simulink model "atrias_boom_nmStand_fullCtrl"  (R2015a)
settings: Solver=ode23t  StartTime=0.0  StopTime=t_end  FixedStep=0.001  MaxStep=1e-3  RelTol=1e-3
InitFcn:
  | addpath('../common/')
  | colors
StartFcn:
  | tic
StopFcn:
  | %stopscript
values from neighbouring files (symbols this model uses):
  A1_notch_f1 = -2*cos(fnotch_f1*sample_time)    [set_control_params.m]
  A2_notch_f1 = 1    [set_control_params.m]
  A_lpf_dtau = 1 + B1_lpf_dtau + B2_lpf_dtau    [set_control_params.m]
  ankle_stiffness = 1/2*pi    (= 1.57079632679)    [mechanical_params.m]
  B1_lpf_dtau = -2*exp(-lpf_damping*fcut_dtau*sample_time)*cos(fcut_dtau*sample_time*sqrt(1-lpf_damping^2))    [set_control_params.m]
  B1_notch_f1 = -2*exp(-notch_damping*fnotch_f1*sample_time)*cos(fnotch_f1*sample_time*sqrt(1-notch_damping^2))    [set_control_params.m]
  B2_lpf_dtau = exp(-2*lpf_damping*fcut_dtau*sample_time)    [set_control_params.m]
  B2_notch_f1 = exp(-2*notch_damping*fnotch_f1*sample_time)    [set_control_params.m]
  b_hmotor = 0    [mechanical_params.m]
  b_leg_spring = 0.075*sqrt(k_leg_spring*0.5*.25^2)    [mechanical_params.m]
  b_rotor = 0*60/(2*pi)*9.725e-5    (= 0)    [mechanical_params.m]
  boom_mount_to_center_diagonal = boom_mount_to_center / cos(pitch_mount_angle)    [mechanical_params.m]    (also in set_control_params.m)
  breakaway_friction = [25 25 25 25]    [mechanical_params.m]
  contactThr = 0.35    [set_control_params.m]
  coulomb_friction = [20 20 20 20]    [mechanical_params.m]
  d_com = (d_hip_com_to_torso_com*m_torso)/(m_torso + num_legs*m_hshaft)    [mechanical_params.m]
  delta_phi_max = 160*pi/180    (= 2.79252680319)    [mechanical_params.m]    (also in set_control_params.m)
  delta_phi_max_buffer = 20*pi/180    (= 0.349065850399)    [set_control_params.m]
  delta_phi_max_dropoff = 2*pi/180    (= 0.0349065850399)    [set_control_params.m]
  delta_phi_min = 25.5*pi/180    (= 0.445058959259)    [mechanical_params.m]    (also in set_control_params.m)
  friction_linear_zone = [0.5 0.5 0.5 0.5].*pi/180    [mechanical_params.m]
  g = 9.803    [mechanical_params.m]    (also in set_control_params.m = 9.81)
  gain_nodes_sea_torque = [0,65,350,700]    [set_control_params.m]
  HIP_MTR_MAX_CONT_TORQUE = HIP_MTR_MAX_CONT_CURRENT*HIP_MOTOR_CONSTANT*HIP_MTR_GEAR_RATIO    (= 86.0016)    [set_control_params.m]
  HIP_MTR_MAX_TORQUE = max_current_hip*Kt_hip*N_h    (= 629.28)    [mechanical_params.m]
  initial_boom_pitch = 0    [mechanical_params.m]
  initial_boom_roll = asin((initial_com_height + boom_mount_to_com + boom_mount_to_center*tan(pitch_mount_angle) - (base_12(2) + yshaft_12(2))) / (l_boom + boom_mount_to_center_diagonal))    [mechanical_params.m]
  initial_boom_yaw = 0    [mechanical_params.m]
  initial_hip_roll = 0*pi/180    (= 0)    [mechanical_params.m]
  initial_winch_angle = -12 * pi/180    (= -0.209439510239)    [mechanical_params.m]
  k_gn = m_total*g/0.01    (= 57041.421916)    [mechanical_params.m]
  k_gt = m_total*g/0.1    (= 5704.1421916)    [mechanical_params.m]
  k_leg_spring = 4118.3    [mechanical_params.m]    (also in set_control_params.m)
  K_notch_f1 = (1+B1_notch_f1+B2_notch_f1)/(1+A1_notch_f1+A2_notch_f1)    [set_control_params.m]
  k_phi = 5000    [mechanical_params.m]
  k_sea = [4118.3 4118.3 4118.3 4118.3]    [set_control_params.m]
  Kb_leg = 0.121    [mechanical_params.m]
  kd_boom_roll_Ctrl = 0    [main_1_nmStand.m]    (also in main_2_nmStand_moveBoom.m)
  kd_lateral = 2*sqrt(kp_lateral*0.8)    [set_control_params.m]
  kd_shin_max = kd_pd_avoid_limits    (= 1000)    [set_control_params.m]
  kd_shin_min = kd_pd_avoid_limits    (= 1000)    [set_control_params.m]
  kd_splay_max = kd_pd_avoid_limits    (= 1000)    [set_control_params.m]
  kd_splay_min = kd_pd_avoid_limits    (= 1000)    [set_control_params.m]
  kd_thigh_max = kd_pd_avoid_limits    (= 1000)    [set_control_params.m]
  kd_thigh_min = kd_pd_avoid_limits    (= 1000)    [set_control_params.m]
  kd_winch = td_winch*kp_winch    (= 989.239577798)    [mechanical_params.m]
  kp_boom_roll_Ctrl = 0    [main_1_nmStand.m]    (also in main_2_nmStand_moveBoom.m)
  kp_lateral = 1000    [set_control_params.m]
  kp_sea_torque = [0.3, 0.3, 6.0, 6.0]    [set_control_params.m]
  kp_shin_max = kp_pd_avoid_limits    (= 5000)    [set_control_params.m]
  kp_shin_min = kp_pd_avoid_limits    (= 5000)    [set_control_params.m]
  kp_splay_max = kp_pd_avoid_limits    (= 5000)    [set_control_params.m]
  kp_splay_min = kp_pd_avoid_limits/10    (= 500)    [set_control_params.m]
  kp_thigh_max = kp_pd_avoid_limits    (= 5000)    [set_control_params.m]
  kp_thigh_min = kp_pd_avoid_limits    (= 5000)    [set_control_params.m]
  kp_winch = winch_gravity_comp/(3*pi/180)    (= 19784.791556)    [mechanical_params.m]
  Kt_leg = 0.121    [mechanical_params.m]
  l_boom = 1.8161    [mechanical_params.m]    (also in set_control_params.m)
  L_leg = 0.102e-3    (= 0.000102)    [mechanical_params.m]
  l_seg = 0.5    [mechanical_params.m]    (also in set_control_params.m)
  l_v = l_seg*cos(min_splay_angle/2)    [set_control_params.m]
  lateral_offset = 0.2    [set_control_params.m]
  lateral_target_angle_right = -6*pi/180    (= -0.10471975512)    [set_control_params.m]
  lateral_transition_force = 150    [set_control_params.m]
  LEG_MTR_MAX_TORQUE = max_current_leg * Kt_leg * N    (= 1210)    [mechanical_params.m]
  loaded_unloaded_torque_threshold = 65*ones(1,4)    [set_control_params.m]
  lowerleg_12 = 0.40    (= 0.4)    [mechanical_params.m]
  m_boom = 4.49    [mechanical_params.m]
  m_fblink = 0.46    [mechanical_params.m]    (also in set_control_params.m)
  m_foot = 0.0857    [mechanical_params.m]
  m_hshaft = 18    [mechanical_params.m]    (also in set_control_params.m = 20)
  m_leg = m_thigh + m_lowerleg + m_shin + m_fblink    (= 2.3438)    [mechanical_params.m]
  m_leg_motor = 18    [set_control_params.m]
  m_lowerleg = 0.4438    [mechanical_params.m]    (also in set_control_params.m)
  m_output_gear = 1e-5    (= 1e-05)    [mechanical_params.m]    (also in set_control_params.m)
  m_rotor = 1e-5    (= 1e-05)    [mechanical_params.m]    (also in set_control_params.m)
  m_shin = 0.75    [mechanical_params.m]    (also in set_control_params.m)
  m_thigh = 0.69    [mechanical_params.m]    (also in set_control_params.m)
  m_torso = 17.5    [mechanical_params.m]    (also in set_control_params.m = 17.9)
  m_total = num_legs*(m_hshaft + m_thigh + m_lowerleg + m_shin + m_fblink + 2*m_gearing) + m_torso    (= 58.18772)    [mechanical_params.m]    (also in set_control_params.m = 62.58772)
  m_virtual_gear = 1e-5    (= 1e-05)    [mechanical_params.m]    (also in set_control_params.m)
  m_yshaft = 12.89    [mechanical_params.m]
  max_current_leg = 200    [mechanical_params.m]
  max_sagittal_loaded_torque = 833    [set_control_params.m]
  max_sagittal_unloaded_torque = 267    [set_control_params.m]
  max_torque_lateral = min(MTR_HIP_MAX_CURRENT, HIP_CURRENT_LIMIT)*HIP_MOTOR_CONSTANT*HIP_MTR_GEAR_RATIO    [set_control_params.m]
  max_voltage_leg = 50    [mechanical_params.m]
  maximum_lateral_angle = 18*pi/180    (= 0.314159265359)    [set_control_params.m]
  min_splay_angle = 45*pi/180    (= 0.785398163397)    [set_control_params.m]
  min_splay_buffer = 1*pi/180    (= 0.0174532925199)    [set_control_params.m]
  min_splay_dropoff = 5*pi/180    (= 0.0872664625997)    [set_control_params.m]
  minimum_lateral_angle = -9.5*pi/180    (= -0.165806278939)    [set_control_params.m]
  mu_hmotor = 0.90    (= 0.9)    [mechanical_params.m]
  mu_motor = 0.85    [mechanical_params.m]
  mu_slide = 0.8    [mechanical_params.m]
  mu_stick = 0.9    [mechanical_params.m]
  N = 50    [mechanical_params.m]
  N_h = r_hip_shaft / r_hip_gearhead    (= 57)    [mechanical_params.m]
  phi_max_collision = -5*pi/180    (= -0.0872664625997)    [mechanical_params.m]
  phi_roll_max = pi + 16*pi/180    (= 3.42084533391)    [mechanical_params.m]
  phi_roll_min = pi - 9*pi/180    (= 2.98451302091)    [mechanical_params.m]
  phi_shin_max = 3*pi/2 + 17.5*pi/180    (= 5.01782159948)    [mechanical_params.m]    (also in set_control_params.m)
  phi_shin_max_buffer = 20*pi/180    (= 0.349065850399)    [set_control_params.m]
  phi_shin_max_dropoff = 2*pi/180    (= 0.0349065850399)    [set_control_params.m]
  phi_shin_min = pi - 45*pi/180    (= 2.35619449019)    [mechanical_params.m]    (also in set_control_params.m)
  phi_shin_min_buffer = 20*pi/180    (= 0.349065850399)    [set_control_params.m]
  phi_shin_min_dropoff = 2*pi/180    (= 0.0349065850399)    [set_control_params.m]
  phi_thigh_max = pi + 45*pi/180    (= 3.92699081699)    [mechanical_params.m]    (also in set_control_params.m)
  phi_thigh_max_buffer = 20*pi/180    (= 0.349065850399)    [set_control_params.m]
  phi_thigh_max_dropoff = 2*pi/180    (= 0.0349065850399)    [set_control_params.m]
  phi_thigh_min = pi/2 - 17.5*pi/180    (= 1.2653637077)    [mechanical_params.m]    (also in set_control_params.m)
  phi_thigh_min_buffer = 20*pi/180    (= 0.349065850399)    [set_control_params.m]
  phi_thigh_min_dropoff = 2*pi/180    (= 0.0349065850399)    [set_control_params.m]
  r_hip_gearhead = 0.009525    [mechanical_params.m]
  r_hip_shaft = 0.542925    [mechanical_params.m]
  R_leg = 0.052    [mechanical_params.m]
  r_rotor = 0.001    [mechanical_params.m]
  r_virtual_gear = N*r_rotor    (= 0.05)    [mechanical_params.m]
  releaseThr = 0.2    [set_control_params.m]
  sample_time = 0.001    [set_control_params.m]
  ... (+19 more)
undefined symbols (not defined in the file or in its folder): A_lpf_velocity, B1_lpf_velocity, B2_lpf_velocity, base_color_d, boom_color_d, c, c_jointstop, CtrlPar_theta0, eref, fblink_color_d, floor_color_d, FmaxBFSH, FmaxGLU, FmaxHAM, FmaxHFL, FmaxRF, FmaxVAS, foot_color_d, FPCtrlPar, hshaft_color_d, j_motor, K, lateral_motor_efficiency, LLCtrlPar, loptBFSH, loptGLU, loptHAM, loptHFL, loptRF, loptVAS, lowerleg_color_d, lslackBFSH, lslackGLU, lslackHAM, lslackHFL, lslackRF, lslackVAS, MidDelay_discrete, Newton, output_sample_time, phi12_max, phi12_min, phi23_max, phi23_min, phimaxRFk, phimaxVAS, phirefBFSH, phirefGLU, phirefHAMh, phirefHAMk, phirefHFL, phirefRFh, phirefRFk, phirefVAS, phiScaleRFk, phiScaleVAS, rad ... (+40)
libraries: sm_lib x210, nesl_utility x140, simulink x58, simulink_extras x26, fl_lib x16, mblibv1 x2, commnoisgen2 x1
(part 15 of 19)

== system atrias_boom_nmStand_fullCtrl/Mechanical System Layer/Ground Contact Models/R Back Ground Contact/3D Contact/Static Friction Model ==
  note: Stiction Limit Detector
  note: Static Friction Model
  note: Zero multiplication prevents
      | horizontal friction model from
      | oscillating between static and kinetic
      | friction when the vertical force is zero but
      | the ground level is not yet reached
      | in the upward motion
  note: (distance to
      | surface)
  note: Tangential Ground Reaction Force
  pos [m] : Inport
  vel [m/s m/s m/s] : Inport  Port=2
  RefPtFP [m m m] : Inport  Port=3
  posFP [m] : Inport  Port=4
  nVecFP [m m m] : Inport  Port=5
  Enable : EnablePort  StatesWhenEnabling=reset  ZeroCross=off
  Abs : Abs
  Check Vertical Friction : Product  RndMeth=Zero
  Constant : Constant
  Dpos_n : DotProduct  InputSameDT=on  OutDataTypeStr=Inherit: Inherit via internal rule
  Dpos_nVec : Product  RndMeth=Zero
  Dpos_tVec : Sum  Inputs=|+-
  FixPt Relational Operator : RelationalOperator  Operator=>  OutDataTypeStr=boolean  ZeroCross=off
  Gain : Gain  Gain=-1
  Gain1 : Gain  Gain=k_gn
  Gain2 : Gain  Gain=1/v_gn_max
  Gain3 : Gain  Gain=k_gt
  Gain5 : Gain  Gain=1/v_gt_max
  Memory : Memory
  Mux2 : Mux  Inputs=2
  Normal Ground Reaction Force : Fcn  Expr="u(1)  *  (1-u(2)) * (u(2)<1)"
  Positive : simulink/Logic and Bit Operations/Compare To Zero  relop=>  OutDataTypeStr=boolean
  Positive1 : simulink/Logic and Bit Operations/Compare To Zero  relop=>  OutDataTypeStr=boolean
  Product1 : Product  RndMeth=Zero
  Sign : Signum  ZeroCross=off
  Sum : Sum  Inputs=-+
  Sum1 : Sum  Inputs=|+-
  Sum2 : Sum  Inputs=|+-
  Vector Norm : Subsystem
  d_n : DotProduct  InputSameDT=on  OutDataTypeStr=Inherit: Inherit via internal rule
  stiction limit force : Gain  Gain=mu_stick
  sum : Sum  Inputs=++|
  tVec1 : Product  Inputs=**  RndMeth=Zero
  tVec2 : Product  Inputs=**  RndMeth=Zero
  v_n : DotProduct  InputSameDT=on  OutDataTypeStr=Inherit: Inherit via internal rule
  v_nVec : Product  RndMeth=Zero
  v_tVec : Sum  Inputs=-+|
  F_n Stick [N N N] : Outport  OutputWhenDisabled=reset  InitialOutput=[0 0 0]
      settings: AttributesFormatString=initial = '%<InitialOutput>'\nwhen disabled = '%<OutputWhenDisabled>'
  F_t Stick [N N N] : Outport  Port=2  OutputWhenDisabled=reset  InitialOutput=[0 0 0]
      settings: AttributesFormatString=when disabled: %<OutputWhenDisabled>\ninitial: %<InitialOutput>
  Sliding! : Outport  Port=3  OutputWhenDisabled=reset  InitialOutput=0
      settings: AttributesFormatString=when disabled: %<OutputWhenDisabled>\ninitial: %<InitialOutput>
  wires:
  Sum/1 -> Positive/1
  Memory/1 -> FixPt Relational Operator/2
  Positive/1 -> FixPt Relational Operator/1, Memory/1
  FixPt Relational Operator/1 -> Sliding!/1
  Abs/1 -> Sum/1
  stiction limit force/1 -> Abs/1
  Positive1/1 -> Check Vertical Friction/2
  Check Vertical Friction/1 -> Vector Norm/1(vec), F_t Stick [N N N]/1
  Normal Ground Reaction Force/1 -> Product1/2, stiction limit force/1, Positive1/1
  Mux2/1 -> Normal Ground Reaction Force/1
  Gain1/1 -> Mux2/1
  Gain2/1 -> Mux2/2
  nVecFP [m m m]/1 -> d_n/1, v_n/2, Dpos_n/1, Dpos_nVec/1, v_nVec/2, Product1/1
  d_n/1 -> Gain1/1
  vel [m/s m/s m/s]/1 -> v_tVec/2, v_n/1
  v_n/1 -> v_nVec/1, Gain2/1
  v_nVec/1 -> v_tVec/1
  v_tVec/1 -> Gain5/1
  Product1/1 -> F_n Stick [N N N]/1
  pos [m]/1 -> Sum2/1, Sum1/2
  posFP [m]/1 -> Sum2/2
  Sum2/1 -> Dpos_n/2, Dpos_tVec/1  "Dpos"
  Dpos_n/1 -> Dpos_nVec/2
  Dpos_nVec/1 -> Dpos_tVec/2
  Dpos_tVec/1 -> Gain3/1
  Gain3/1 -> Sign/1, tVec2/2
  Sign/1 -> tVec1/2
  tVec1/1 -> sum/2
  Constant/1 -> sum/1
  sum/1 -> tVec2/1
  tVec2/1 -> Gain/1
  Gain/1 -> Check Vertical Friction/1
  Vector Norm/1(norm) -> Sum/2
  RefPtFP [m m m]/1 -> Sum1/1
  Sum1/1 -> d_n/2
  Gain5/1 -> tVec1/1

== system atrias_boom_nmStand_fullCtrl/Mechanical System Layer/Ground Contact Models/R Front Ground Contact/3D Contact/Friction Switch ==
  note: Static/Kinetic Friction Switch
  Slide! : Inport
  Stick! : Inport  Port=2
  Memory : Memory
  S-R Flip-Flop : simulink_extras/Flip Flops/S-R Flip-Flop  initial_condition=0
  Terminator : Terminator
  Stiction : Outport
  wires:
  S-R Flip-Flop/1 -> Memory/1
  S-R Flip-Flop/2 -> Terminator/1
  Stick!/1 -> S-R Flip-Flop/1
  Slide!/1 -> S-R Flip-Flop/2
  Memory/1 -> Stiction/1

== system atrias_boom_nmStand_fullCtrl/Mechanical System Layer/Ground Contact Models/R Front Ground Contact/3D Contact/Kinetic Friction Model ==
  note: Kinetic Friction Model
  note: Footpoint Determiner
  note: Sliding Limit Detector
  note: Normal Ground Friction
  note: Tangential Ground Friction
  vel [m/s m/s m/s] : Inport
  pos [m m m] : Inport  Port=2
  RefPt [m m m] : Inport  Port=3
  nVec [m m m] : Inport  Port=4
  Enable : EnablePort  StatesWhenEnabling=reset  ZeroCross=off
  Constant : Constant  Value=vLimit
  Constant1 : Constant  Value=[0 0 0 1]'
  Demux : Demux  Outputs=[3 1]
  FixPt Relational Operator : RelationalOperator  Operator=>  OutDataTypeStr=boolean  ZeroCross=off
  Gain3 : Gain  Gain=k_gn
  Gain4 : Gain  Gain=1/v_gn_max
  Memory : Memory
  Mux1 : Mux  Inputs=2
  Mux2 : Mux  Inputs=2
  Negative : simulink/Logic and Bit Operations/Compare To Zero  relop=<  OutDataTypeStr=boolean
  Normal Axis Ground Force : Fcn  Expr="u(1)  *  (1-u(2)) * (u(2)<1)"
  Product : Product  RndMeth=Zero
  Product1 : Product  RndMeth=Zero
  Sum : Sum  Inputs=|+-
  Switch : Switch  Criteria=u2 > Threshold  Threshold=0.9*vLimit
      settings: AttributesFormatString=>%<Threshold>?
  Vector Norm : Subsystem
  d_n : DotProduct  InputSameDT=on  OutDataTypeStr=Inherit: Inherit via internal rule
  qnVec : Sum  Inputs=-+
  reverse direction : Gain  Gain=-1
  sliding friction coefficient : Gain  Gain=mu_slide
  tVec : Product  Inputs=*/  RndMeth=Zero
  v_n : DotProduct  InputSameDT=on  OutDataTypeStr=Inherit: Inherit via internal rule
  v_nVec : Product  RndMeth=Zero
  v_tVec : Sum  Inputs=-+|
  RefPtFP [m m m] : Outport  InitialOutput=[0 0 0]
      settings: AttributesFormatString=initial = '%<InitialOutput>'\nwhen disabled = '%<OutputWhenDisabled>'
  posFP [m m m] : Outport  Port=2  InitialOutput=[0 0 0]
      settings: AttributesFormatString=initial = '%<InitialOutput>'\nwhen disabled = '%<OutputWhenDisabled>'
  nVec FP [m m m] : Outport  Port=3  InitialOutput=0
      settings: AttributesFormatString=initial = '%<InitialOutput>'\nwhen disabled = '%<OutputWhenDisabled>'
  Stiction! : Outport  Port=4  OutputWhenDisabled=reset  InitialOutput=0
      settings: AttributesFormatString=initial = '%<InitialOutput>'\nwhen disabled = '%<OutputWhenDisabled>'
  F_t Slide [N N N] : Outport  Port=5  OutputWhenDisabled=reset  InitialOutput=[0 0 0]
      settings: AttributesFormatString=initial = '%<InitialOutput>'\nwhen disabled = '%<OutputWhenDisabled>'
  F_n Slide [N N N] : Outport  Port=6  OutputWhenDisabled=reset  InitialOutput=[0 0 0]
      settings: AttributesFormatString=initial = '%<InitialOutput>'\nwhen disabled = '%<OutputWhenDisabled>'
  wires:
  Normal Axis Ground Force/1 -> sliding friction coefficient/1, Product1/2
  Product/1 -> F_t Slide [N N N]/1
  FixPt Relational Operator/1 -> Stiction!/1
  Memory/1 -> FixPt Relational Operator/2
  Negative/1 -> FixPt Relational Operator/1, Memory/1
  Vector Norm/1(norm) -> Sum/1, Switch/2, Mux2/2
  Sum/1 -> Negative/1
  Constant/1 -> Sum/2
  Mux1/1 -> Normal Axis Ground Force/1
  Gain3/1 -> Mux1/1
  Gain4/1 -> Mux1/2
  nVec [m m m]/1 -> v_n/1, v_nVec/2, d_n/2, Product1/1, nVec FP [m m m]/1
  d_n/1 -> Gain3/1
  vel [m/s m/s m/s]/1 -> v_n/2, v_tVec/2
  v_n/1 -> Gain4/1, v_nVec/1
  v_nVec/1 -> v_tVec/1
  v_tVec/1 -> Vector Norm/1(vec), Mux2/1
  sliding friction coefficient/1 -> Product/1
  reverse direction/1 -> Product/2
  Product1/1 -> F_n Slide [N N N]/1
  tVec/1 -> reverse direction/1
  Constant1/1 -> Switch/3
  Mux2/1 -> Switch/1
  Switch/1 -> Demux/1
  Demux/2 -> tVec/2
  Demux/1 -> tVec/1
  pos [m m m]/1 -> posFP [m m m]/1, qnVec/1
  qnVec/1 -> d_n/1
  RefPt [m m m]/1 -> qnVec/2, RefPtFP [m m m]/1

== system atrias_boom_nmStand_fullCtrl/Mechanical System Layer/Ground Contact Models/R Front Ground Contact/3D Contact/Static Friction Model ==
  note: Stiction Limit Detector
  note: Static Friction Model
  note: Zero multiplication prevents
      | horizontal friction model from
      | oscillating between static and kinetic
      | friction when the vertical force is zero but
      | the ground level is not yet reached
      | in the upward motion
  note: (distance to
      | surface)
  note: Tangential Ground Reaction Force
  pos [m] : Inport
  vel [m/s m/s m/s] : Inport  Port=2
  RefPtFP [m m m] : Inport  Port=3
  posFP [m] : Inport  Port=4
  nVecFP [m m m] : Inport  Port=5
  Enable : EnablePort  StatesWhenEnabling=reset  ZeroCross=off
  Abs : Abs
  Check Vertical Friction : Product  RndMeth=Zero
  Constant : Constant
  Dpos_n : DotProduct  InputSameDT=on  OutDataTypeStr=Inherit: Inherit via internal rule
  Dpos_nVec : Product  RndMeth=Zero
  Dpos_tVec : Sum  Inputs=|+-
  FixPt Relational Operator : RelationalOperator  Operator=>  OutDataTypeStr=boolean  ZeroCross=off
  Gain : Gain  Gain=-1
  Gain1 : Gain  Gain=k_gn
  Gain2 : Gain  Gain=1/v_gn_max
  Gain3 : Gain  Gain=k_gt
  Gain5 : Gain  Gain=1/v_gt_max
  Memory : Memory
  Mux2 : Mux  Inputs=2
  Normal Ground Reaction Force : Fcn  Expr="u(1)  *  (1-u(2)) * (u(2)<1)"
  Positive : simulink/Logic and Bit Operations/Compare To Zero  relop=>  OutDataTypeStr=boolean
  Positive1 : simulink/Logic and Bit Operations/Compare To Zero  relop=>  OutDataTypeStr=boolean
  Product1 : Product  RndMeth=Zero
  Sign : Signum  ZeroCross=off
  Sum : Sum  Inputs=-+
  Sum1 : Sum  Inputs=|+-
  Sum2 : Sum  Inputs=|+-
  Vector Norm : Subsystem
  d_n : DotProduct  InputSameDT=on  OutDataTypeStr=Inherit: Inherit via internal rule
  stiction limit force : Gain  Gain=mu_stick
  sum : Sum  Inputs=++|
  tVec1 : Product  Inputs=**  RndMeth=Zero
  tVec2 : Product  Inputs=**  RndMeth=Zero
  v_n : DotProduct  InputSameDT=on  OutDataTypeStr=Inherit: Inherit via internal rule
  v_nVec : Product  RndMeth=Zero
  v_tVec : Sum  Inputs=-+|
  F_n Stick [N N N] : Outport  OutputWhenDisabled=reset  InitialOutput=[0 0 0]
      settings: AttributesFormatString=initial = '%<InitialOutput>'\nwhen disabled = '%<OutputWhenDisabled>'
  F_t Stick [N N N] : Outport  Port=2  OutputWhenDisabled=reset  InitialOutput=[0 0 0]
      settings: AttributesFormatString=when disabled: %<OutputWhenDisabled>\ninitial: %<InitialOutput>
  Sliding! : Outport  Port=3  OutputWhenDisabled=reset  InitialOutput=0
      settings: AttributesFormatString=when disabled: %<OutputWhenDisabled>\ninitial: %<InitialOutput>
  wires:
  Sum/1 -> Positive/1
  Memory/1 -> FixPt Relational Operator/2
  Positive/1 -> FixPt Relational Operator/1, Memory/1
  FixPt Relational Operator/1 -> Sliding!/1
  Abs/1 -> Sum/1
  stiction limit force/1 -> Abs/1
  Positive1/1 -> Check Vertical Friction/2
  Check Vertical Friction/1 -> Vector Norm/1(vec), F_t Stick [N N N]/1
  Normal Ground Reaction Force/1 -> Product1/2, stiction limit force/1, Positive1/1
  Mux2/1 -> Normal Ground Reaction Force/1
  Gain1/1 -> Mux2/1
  Gain2/1 -> Mux2/2
  nVecFP [m m m]/1 -> d_n/1, v_n/2, Dpos_n/1, Dpos_nVec/1, v_nVec/2, Product1/1
  d_n/1 -> Gain1/1
  vel [m/s m/s m/s]/1 -> v_tVec/2, v_n/1
  v_n/1 -> v_nVec/1, Gain2/1
  v_nVec/1 -> v_tVec/1
  v_tVec/1 -> Gain5/1
  Product1/1 -> F_n Stick [N N N]/1
  pos [m]/1 -> Sum2/1, Sum1/2
  posFP [m]/1 -> Sum2/2
  Sum2/1 -> Dpos_n/2, Dpos_tVec/1  "Dpos"
  Dpos_n/1 -> Dpos_nVec/2
  Dpos_nVec/1 -> Dpos_tVec/2
  Dpos_tVec/1 -> Gain3/1
  Gain3/1 -> Sign/1, tVec2/2
  Sign/1 -> tVec1/2
  tVec1/1 -> sum/2
  Constant/1 -> sum/1
  sum/1 -> tVec2/1
  tVec2/1 -> Gain/1
  Gain/1 -> Check Vertical Friction/1
  Vector Norm/1(norm) -> Sum/2
  RefPtFP [m m m]/1 -> Sum1/1
  Sum1/1 -> d_n/2
  Gain5/1 -> tVec1/1

== system atrias_boom_nmStand_fullCtrl/Mechanical System Layer/L Leg/Shin SEA/Rotor and Gearing/Rotational Simscape Intf ==
  Ideal Angular Velocity Source : fl_lib/Mechanical/Mechanical Sources/Ideal Angular Velocity Source
  Ideal Torque Sensor : fl_lib/Mechanical/Mechanical Sensors/Ideal Torque Sensor
  w : PMIOPort  Port=1  Side=Left
  T : PMIOPort  Port=2  Side=Right
  R : PMIOPort  Port=3  Side=Left
  C : PMIOPort  Port=4  Side=Right
  connections:
  Ideal Torque Sensor/RConn1 -- C/RConn1
  R/RConn1 -- Ideal Angular Velocity Source/LConn1
  Ideal Torque Sensor/LConn1 -- Ideal Angular Velocity Source/RConn2
  T/RConn1 -- Ideal Torque Sensor/RConn2
  w/RConn1 -- Ideal Angular Velocity Source/RConn1

== system atrias_boom_nmStand_fullCtrl/Mechanical System Layer/L Leg/Thigh SEA/Rotor and Gearing/Rotational Simscape Intf ==
  Ideal Angular Velocity Source : fl_lib/Mechanical/Mechanical Sources/Ideal Angular Velocity Source
  Ideal Torque Sensor : fl_lib/Mechanical/Mechanical Sensors/Ideal Torque Sensor
  w : PMIOPort  Port=1  Side=Left
  T : PMIOPort  Port=2  Side=Right
  R : PMIOPort  Port=3  Side=Left
  C : PMIOPort  Port=4  Side=Right
  connections:
  Ideal Torque Sensor/RConn1 -- C/RConn1
  R/RConn1 -- Ideal Angular Velocity Source/LConn1
  Ideal Torque Sensor/LConn1 -- Ideal Angular Velocity Source/RConn2
  T/RConn1 -- Ideal Torque Sensor/RConn2
  w/RConn1 -- Ideal Angular Velocity Source/RConn1

== system atrias_boom_nmStand_fullCtrl/Mechanical System Layer/R Leg/Shin SEA/Rotor and Gearing/Rotational Simscape Intf ==
  Ideal Angular Velocity Source : fl_lib/Mechanical/Mechanical Sources/Ideal Angular Velocity Source
  Ideal Torque Sensor : fl_lib/Mechanical/Mechanical Sensors/Ideal Torque Sensor
  w : PMIOPort  Port=1  Side=Left
  T : PMIOPort  Port=2  Side=Right
  R : PMIOPort  Port=3  Side=Left
  C : PMIOPort  Port=4  Side=Right
  connections:
  Ideal Torque Sensor/RConn1 -- C/RConn1
  R/RConn1 -- Ideal Angular Velocity Source/LConn1
  Ideal Torque Sensor/LConn1 -- Ideal Angular Velocity Source/RConn2
  T/RConn1 -- Ideal Torque Sensor/RConn2
  w/RConn1 -- Ideal Angular Velocity Source/RConn1

== system atrias_boom_nmStand_fullCtrl/Mechanical System Layer/R Leg/Thigh SEA/Rotor and Gearing/Rotational Simscape Intf ==
  Ideal Angular Velocity Source : fl_lib/Mechanical/Mechanical Sources/Ideal Angular Velocity Source
  Ideal Torque Sensor : fl_lib/Mechanical/Mechanical Sensors/Ideal Torque Sensor
  w : PMIOPort  Port=1  Side=Left
  T : PMIOPort  Port=2  Side=Right
  R : PMIOPort  Port=3  Side=Left
  C : PMIOPort  Port=4  Side=Right
  connections:
  Ideal Torque Sensor/RConn1 -- C/RConn1
  R/RConn1 -- Ideal Angular Velocity Source/LConn1
  Ideal Torque Sensor/LConn1 -- Ideal Angular Velocity Source/RConn2
  T/RConn1 -- Ideal Torque Sensor/RConn2
  w/RConn1 -- Ideal Angular Velocity Source/RConn1

== system atrias_boom_nmStand_fullCtrl/Control/Behavior Control/Add Limit Avoidance PD Torques/mechanical limit avoidance/PD Joint Limit/L Scale desired torque ==
  note: NOTE: min_splay_angle does not equal delta_phi_min
  phi_thigh [rad] : Inport
  phi_shin [rad] : Inport  Port=2
  Constant : Constant
  Constant1 : Constant  Value=delta_phi_max - delta_phi_max_buffer
  Constant10 : Constant  Value=phi_thigh_max_dropoff
  Constant11 : Constant  Value=phi_shin_min_dropoff
  Constant12 : Constant  Value=phi_shin_max_dropoff
  Constant13 : Constant
  Constant2 : Constant  Value=phi_thigh_max - phi_thigh_max_buffer
  Constant3 : Constant  Value=min_splay_angle+min_splay_buffer
  Constant4 : Constant  Value=phi_thigh_min + phi_thigh_min_buffer
  Constant5 : Constant  Value=phi_shin_max - phi_shin_max_buffer
  Constant6 : Constant  Value=phi_shin_min + phi_shin_min_buffer
  Constant7 : Constant  Value=min_splay_dropoff
  Constant8 : Constant  Value=delta_phi_max_dropoff
  Constant9 : Constant  Value=phi_thigh_min_dropoff
  Divide{,1..5} (6 alike) : Product  Inputs=/*
  Gain : Gain  Gain=-1
  Gain1 : Gain  Gain=-1
  Gain2 : Gain  Gain=-1
  L PD scale : Scope  NumInputPorts=4
      settings: ShowLegends=on  TimeRange=2.5  YMin=-100~-5e+07~-1e+07~-5  YMax=100~1e+07~5e+07~5  SaveName=ScopeData5
  Mux{,1,7..8} (4 alike) : Mux  Inputs=2
  Sum : Sum  Inputs=|+-
  Sum1 : Sum  Inputs=-+|
  Sum2 : Sum  Inputs=+-
  Sum{3..8} (6 alike) : Sum  Inputs=+-|
  [0,1]{,1..5} (6 alike) : Saturate  UpperLimit=1  LowerLimit=0
  max : MinMax  Function=max  Inputs=4
  max2 : MinMax  Function=max  Inputs=4
  scale_back : Outport
  scale_front : Outport  Port=2
  wires:
  Mux1/1 -> L PD scale/4
  Sum1/1 -> scale_front/1, Mux1/2
  [min_thigh_scale] -> max2/3
  [max_thigh_scale] -> max2/4
  [max_splay_scale] -> max/4, max2/2
  [min_splay_scale] -> max/3, max2/1
  [max_shin_scale] -> max/2
  [min_shin_scale] -> max/1
  max2/1 -> Sum1/1
  Constant13/1 -> Sum1/2
  Gain2/1 -> Divide5/2
  Constant12/1 -> Divide5/1
  Sum7/1 -> Gain2/1
  "[0,1]5"/1 -> [max_shin_scale]
  Divide5/1 -> "[0,1]5"/1
  Constant11/1 -> Divide4/1
  Sum8/1 -> Divide4/2
  "[0,1]4"/1 -> [min_shin_scale]
  Divide4/1 -> "[0,1]4"/1
  Constant10/1 -> Divide3/1
  Sum5/1 -> Gain1/1
  Gain1/1 -> Divide3/2
  "[0,1]3"/1 -> [max_thigh_scale]
  Divide3/1 -> "[0,1]3"/1
  Constant9/1 -> Divide2/1
  Sum6/1 -> Divide2/2
  "[0,1]2"/1 -> [min_thigh_scale]
  Divide2/1 -> "[0,1]2"/1
  Gain/1 -> Divide1/2
  Constant8/1 -> Divide1/1
  Sum3/1 -> Gain/1
  "[0,1]1"/1 -> [max_splay_scale]
  Divide1/1 -> "[0,1]1"/1
  "[0,1]"/1 -> [min_splay_scale]
  Divide/1 -> "[0,1]"/1
  Sum4/1 -> Divide/2
  Constant7/1 -> Divide/1
  max/1 -> Sum/2
  Constant/1 -> Sum/1
  Sum/1 -> scale_back/1, Mux1/1
  [max_splay_scale] -> Mux7/2  "max_splay_trq"
  [min_splay_scale] -> Mux7/1  "min_splay_trq"
  Mux7/1 -> L PD scale/3
  Mux8/1 -> L PD scale/2
  [max_shin_scale] -> Mux8/2  "max_shin_trq"
  [min_shin_scale] -> Mux8/1  "min_shin_trq"
  Mux/1 -> L PD scale/1
  [max_thigh_scale] -> Mux/2  "max_thigh_trq"
  [min_thigh_scale] -> Mux/1  "min_thigh_trq"
  Constant5/1 -> Sum7/1
  [shin] -> Sum7/2
  Constant6/1 -> Sum8/1
  [shin] -> Sum8/2
  Constant2/1 -> Sum5/1
  [thigh] -> Sum5/2
  Constant4/1 -> Sum6/1
  [thigh] -> Sum6/2
  Constant1/1 -> Sum3/1
  [splay] -> Sum3/2
  Constant3/1 -> Sum4/1
  [splay] -> Sum4/2
  Sum2/1 -> [splay]  "splay angle"
  phi_thigh [rad]/1 -> Sum2/2, [thigh]
  phi_shin [rad]/1 -> Sum2/1, [shin]

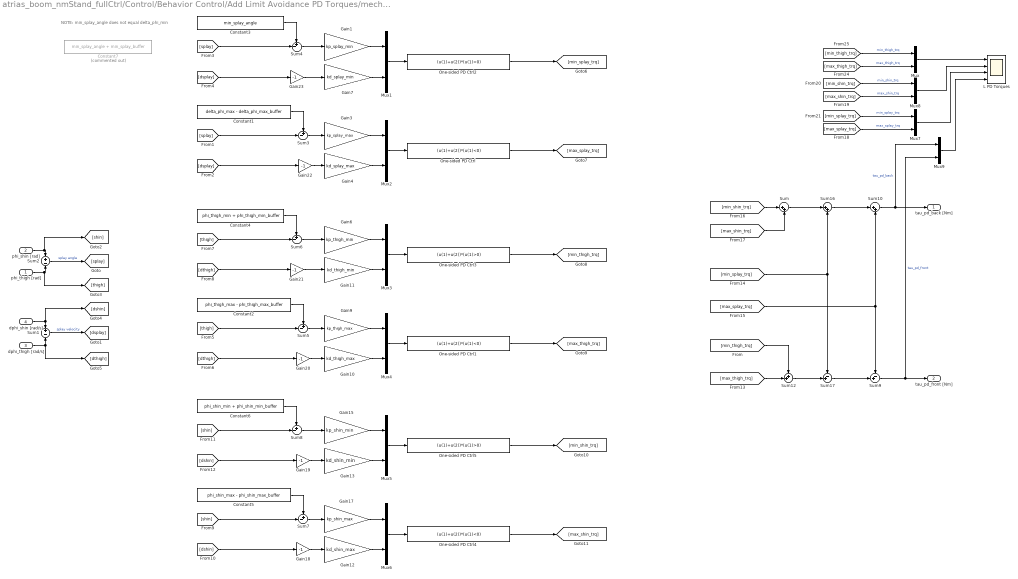
== system atrias_boom_nmStand_fullCtrl/Control/Behavior Control/Add Limit Avoidance PD Torques/mechanical limit avoidance/PD Joint Limit/L mechanical Limit Avoidance Torques (Virtual) ==
  note: NOTE: min_splay_angle does not equal delta_phi_min
  phi_thigh [rad] : Inport
  phi_shin [rad] : Inport  Port=2
  dphi_thigh [rad/s] : Inport  Port=3
  dphi_shin [rad/s] : Inport  Port=4
  Constant1 : Constant  Value=delta_phi_max - delta_phi_max_buffer
  Constant2 : Constant  Value=phi_thigh_max - phi_thigh_max_buffer
  Constant3 : Constant  Value=min_splay_angle
  Constant4 : Constant  Value=phi_thigh_min + phi_thigh_min_buffer
  Constant5 : Constant  Value=phi_shin_max - phi_shin_max_buffer
  Constant6 : Constant  Value=phi_shin_min + phi_shin_min_buffer
  Constant7 : Constant  Commented=on  Value=min_splay_angle + min_splay_buffer
  Gain1 : Gain  Gain=kp_splay_min
  Gain10 : Gain  Gain=kd_thigh_max
  Gain11 : Gain  Gain=kd_thigh_min
  Gain12 : Gain  Gain=kd_shin_max
  Gain13 : Gain  Gain=kd_shin_min
  Gain15 : Gain  Gain=kp_shin_min
  Gain17 : Gain  Gain=kp_shin_max
  Gain{18..23} (6 alike) : Gain  Gain=-1
  Gain3 : Gain  Gain=kp_splay_max
  Gain4 : Gain  Gain=kd_splay_max
  Gain6 : Gain  Gain=kp_thigh_min
  Gain7 : Gain  Gain=kd_splay_min
  Gain9 : Gain  Gain=kp_thigh_max
  L PD Torques : Scope  NumInputPorts=4
      settings: ShowLegends=on  TimeRange=2.5  YMin=-100~-5e+07~-1e+07~-5  YMax=100~1e+07~5e+07~5  SaveName=ScopeData5
  Mux{,1..9} (10 alike) : Mux  Inputs=2
  One-sided PD Ctrl : Fcn  Expr=(u(1)+u(2))*(u(1)<0)
  One-sided PD Ctrl1 : Fcn  Expr=(u(1)+u(2))*(u(1)<0)
  One-sided PD Ctrl2 : Fcn  Expr=(u(1)+u(2))*(u(1)>0)
  One-sided PD Ctrl3 : Fcn  Expr=(u(1)+u(2))*(u(1)>0)
  One-sided PD Ctrl4 : Fcn  Expr=(u(1)+u(2))*(u(1)<0)
  One-sided PD Ctrl5 : Fcn  Expr=(u(1)+u(2))*(u(1)>0)
  Sum : Sum  Inputs=|++
  Sum1 : Sum  Inputs=+-
  Sum10 : Sum  Inputs=|++
  Sum12 : Sum  Inputs=++|
  Sum16 : Sum  Inputs=|++
  Sum17 : Sum  Inputs=-+|
  Sum2 : Sum  Inputs=+-
  Sum{3..8} (6 alike) : Sum  Inputs=+-|
  Sum9 : Sum  Inputs=-+|
  tau_pd_back [Nm] : Outport
  tau_pd_front [Nm] : Outport  Port=2
  wires:
  Mux9/1 -> L PD Torques/4
  dphi_shin [rad/s]/1 -> [dshin], Sum1/1
  dphi_thigh [rad/s]/1 -> [dthigh], Sum1/2
  phi_shin [rad]/1 -> [shin], Sum2/1
  phi_thigh [rad]/1 -> [thigh], Sum2/2
  Sum2/1 -> [splay]  "splay angle"
  Sum1/1 -> [dsplay]  "splay velocity"
  [dsplay] -> Gain23/1
  [splay] -> Sum4/2
  Gain7/1 -> Mux1/2
  Gain1/1 -> Mux1/1
  Sum4/1 -> Gain1/1
  Constant3/1 -> Sum4/1
  Mux1/1 -> One-sided PD Ctrl2/1
  [dsplay] -> Gain22/1
  [splay] -> Sum3/2
  Gain4/1 -> Mux2/2
  Gain3/1 -> Mux2/1
  Sum3/1 -> Gain3/1
  Constant1/1 -> Sum3/1
  Mux2/1 -> One-sided PD Ctrl/1
  [dthigh] -> Gain21/1
  [thigh] -> Sum6/2
  Gain11/1 -> Mux3/2
  Gain6/1 -> Mux3/1
  Sum6/1 -> Gain6/1
  Constant4/1 -> Sum6/1
  Mux3/1 -> One-sided PD Ctrl3/1
  [dthigh] -> Gain20/1
  [thigh] -> Sum5/2
  Gain10/1 -> Mux4/2
  Gain9/1 -> Mux4/1
  Sum5/1 -> Gain9/1
  Constant2/1 -> Sum5/1
  Mux4/1 -> One-sided PD Ctrl1/1
  [dshin] -> Gain19/1
  [shin] -> Sum8/2
  Gain13/1 -> Mux5/2
  Gain15/1 -> Mux5/1
  Sum8/1 -> Gain15/1
  Constant6/1 -> Sum8/1
  Mux5/1 -> One-sided PD Ctrl5/1
  [dshin] -> Gain18/1
  [shin] -> Sum7/2
  Gain12/1 -> Mux6/2
  Gain17/1 -> Mux6/1
  Sum7/1 -> Gain17/1
  Constant5/1 -> Sum7/1
  Mux6/1 -> One-sided PD Ctrl4/1
  One-sided PD Ctrl2/1 -> [min_splay_trq]
  [min_thigh_trq] -> Mux/1  "min_thigh_trq"
  [max_thigh_trq] -> Mux/2  "max_thigh_trq"
  Mux/1 -> L PD Torques/1
  [min_shin_trq] -> Mux8/1  "min_shin_trq"
  [max_shin_trq] -> Mux8/2  "max_shin_trq"
  Mux8/1 -> L PD Torques/2
  Mux7/1 -> L PD Torques/3
  [min_splay_trq] -> Mux7/1  "min_splay_trq"
  [max_splay_trq] -> Mux7/2  "max_splay_trq"
  Sum10/1 -> tau_pd_back [Nm]/1, Mux9/1  "tau_pd_back"
  Sum9/1 -> tau_pd_front [Nm]/1, Mux9/2  "tau_pd_front"
  Sum/1 -> Sum16/1
  [min_shin_trq] -> Sum/1
  [max_shin_trq] -> Sum/2
  Sum16/1 -> Sum10/1
  [min_splay_trq] -> Sum17/1, Sum16/2
  [max_splay_trq] -> Sum9/1, Sum10/2
  [max_thigh_trq] -> Sum12/2
  [min_thigh_trq] -> Sum12/1
  Sum12/1 -> Sum17/2
  Sum17/1 -> Sum9/2
  Gain18/1 -> Gain12/1
  Gain19/1 -> Gain13/1
  Gain20/1 -> Gain10/1
  Gain21/1 -> Gain11/1
  Gain22/1 -> Gain4/1
  Gain23/1 -> Gain7/1
  One-sided PD Ctrl/1 -> [max_splay_trq]
  One-sided PD Ctrl3/1 -> [min_thigh_trq]
  One-sided PD Ctrl1/1 -> [max_thigh_trq]
  One-sided PD Ctrl5/1 -> [min_shin_trq]
  One-sided PD Ctrl4/1 -> [max_shin_trq]

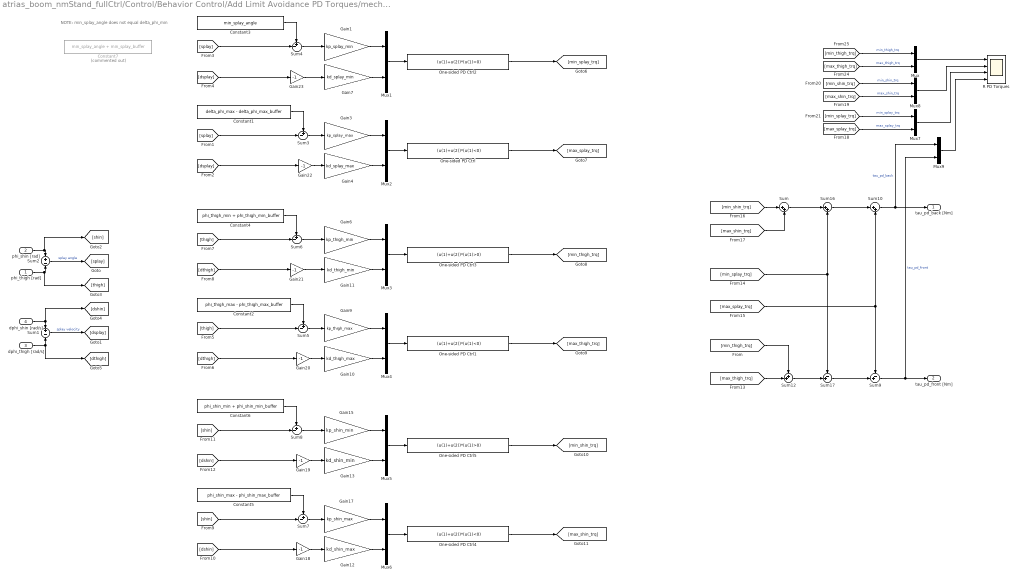
== system atrias_boom_nmStand_fullCtrl/Control/Behavior Control/Add Limit Avoidance PD Torques/mechanical limit avoidance/PD Joint Limit/R Mechanical Limit Avoidance Torques (Virtual)1 ==
  note: NOTE: min_splay_angle does not equal delta_phi_min
  phi_thigh [rad] : Inport
  phi_shin [rad] : Inport  Port=2
  dphi_thigh [rad/s] : Inport  Port=3
  dphi_shin [rad/s] : Inport  Port=4
  Constant1 : Constant  Value=delta_phi_max - delta_phi_max_buffer
  Constant2 : Constant  Value=phi_thigh_max - phi_thigh_max_buffer
  Constant3 : Constant  Value=min_splay_angle
  Constant4 : Constant  Value=phi_thigh_min + phi_thigh_min_buffer
  Constant5 : Constant  Value=phi_shin_max - phi_shin_max_buffer
  Constant6 : Constant  Value=phi_shin_min + phi_shin_min_buffer
  Constant7 : Constant  Commented=on  Value=min_splay_angle + min_splay_buffer
  Gain1 : Gain  Gain=kp_splay_min
  Gain10 : Gain  Gain=kd_thigh_max
  Gain11 : Gain  Gain=kd_thigh_min
  Gain12 : Gain  Gain=kd_shin_max
  Gain13 : Gain  Gain=kd_shin_min
  Gain15 : Gain  Gain=kp_shin_min
  Gain17 : Gain  Gain=kp_shin_max
  Gain{18..23} (6 alike) : Gain  Gain=-1
  Gain3 : Gain  Gain=kp_splay_max
  Gain4 : Gain  Gain=kd_splay_max
  Gain6 : Gain  Gain=kp_thigh_min
  Gain7 : Gain  Gain=kd_splay_min
  Gain9 : Gain  Gain=kp_thigh_max
  Mux{,1..9} (10 alike) : Mux  Inputs=2
  One-sided PD Ctrl : Fcn  Expr=(u(1)+u(2))*(u(1)<0)
  One-sided PD Ctrl1 : Fcn  Expr=(u(1)+u(2))*(u(1)<0)
  One-sided PD Ctrl2 : Fcn  Expr=(u(1)+u(2))*(u(1)>0)
  One-sided PD Ctrl3 : Fcn  Expr=(u(1)+u(2))*(u(1)>0)
  One-sided PD Ctrl4 : Fcn  Expr=(u(1)+u(2))*(u(1)<0)
  One-sided PD Ctrl5 : Fcn  Expr=(u(1)+u(2))*(u(1)>0)
  R PD Torques : Scope  NumInputPorts=4
      settings: ShowLegends=on  TimeRange=2.5  YMin=-100~-5e+07~-1e+07~-5  YMax=100~1e+07~5e+07~5  SaveName=ScopeData5
  Sum : Sum  Inputs=|++
  Sum1 : Sum  Inputs=+-
  Sum10 : Sum  Inputs=|++
  Sum12 : Sum  Inputs=++|
  Sum16 : Sum  Inputs=|++
  Sum17 : Sum  Inputs=-+|
  Sum2 : Sum  Inputs=+-
  Sum{3..8} (6 alike) : Sum  Inputs=+-|
  Sum9 : Sum  Inputs=-+|
  tau_pd_back [Nm] : Outport
  tau_pd_front [Nm] : Outport  Port=2
  wires:
  One-sided PD Ctrl4/1 -> [max_shin_trq]
  One-sided PD Ctrl5/1 -> [min_shin_trq]
  One-sided PD Ctrl1/1 -> [max_thigh_trq]
  One-sided PD Ctrl3/1 -> [min_thigh_trq]
  One-sided PD Ctrl/1 -> [max_splay_trq]
  Gain23/1 -> Gain7/1
  Gain22/1 -> Gain4/1
  Gain21/1 -> Gain11/1
  Gain20/1 -> Gain10/1
  Gain19/1 -> Gain13/1
  Gain18/1 -> Gain12/1
  Sum17/1 -> Sum9/2
  Sum12/1 -> Sum17/2
  [min_thigh_trq] -> Sum12/1
  [max_thigh_trq] -> Sum12/2
  [max_splay_trq] -> Sum10/2, Sum9/1
  [min_splay_trq] -> Sum16/2, Sum17/1
  Sum16/1 -> Sum10/1
  [max_shin_trq] -> Sum/2
  [min_shin_trq] -> Sum/1
  Sum/1 -> Sum16/1
  Sum9/1 -> Mux9/2, tau_pd_front [Nm]/1  "tau_pd_front"
  Sum10/1 -> Mux9/1, tau_pd_back [Nm]/1  "tau_pd_back"
  [max_splay_trq] -> Mux7/2  "max_splay_trq"
  [min_splay_trq] -> Mux7/1  "min_splay_trq"
  Mux7/1 -> R PD Torques/3
  Mux8/1 -> R PD Torques/2
  [max_shin_trq] -> Mux8/2  "max_shin_trq"
  [min_shin_trq] -> Mux8/1  "min_shin_trq"
  Mux/1 -> R PD Torques/1
  [max_thigh_trq] -> Mux/2  "max_thigh_trq"
  [min_thigh_trq] -> Mux/1  "min_thigh_trq"
  One-sided PD Ctrl2/1 -> [min_splay_trq]
  Mux6/1 -> One-sided PD Ctrl4/1
  Constant5/1 -> Sum7/1
  Sum7/1 -> Gain17/1
  Gain17/1 -> Mux6/1
  Gain12/1 -> Mux6/2
  [shin] -> Sum7/2
  [dshin] -> Gain18/1
  Mux5/1 -> One-sided PD Ctrl5/1
  Constant6/1 -> Sum8/1
  Sum8/1 -> Gain15/1
  Gain15/1 -> Mux5/1
  Gain13/1 -> Mux5/2
  [shin] -> Sum8/2
  [dshin] -> Gain19/1
  Mux4/1 -> One-sided PD Ctrl1/1
  Constant2/1 -> Sum5/1
  Sum5/1 -> Gain9/1
  Gain9/1 -> Mux4/1
  Gain10/1 -> Mux4/2
  [thigh] -> Sum5/2
  [dthigh] -> Gain20/1
  Mux3/1 -> One-sided PD Ctrl3/1
  Constant4/1 -> Sum6/1
  Sum6/1 -> Gain6/1
  Gain6/1 -> Mux3/1
  Gain11/1 -> Mux3/2
  [thigh] -> Sum6/2
  [dthigh] -> Gain21/1
  Mux2/1 -> One-sided PD Ctrl/1
  Constant1/1 -> Sum3/1
  Sum3/1 -> Gain3/1
  Gain3/1 -> Mux2/1
  Gain4/1 -> Mux2/2
  [splay] -> Sum3/2
  [dsplay] -> Gain22/1
  Mux1/1 -> One-sided PD Ctrl2/1
  Constant3/1 -> Sum4/1
  Sum4/1 -> Gain1/1
  Gain1/1 -> Mux1/1
  Gain7/1 -> Mux1/2
  [splay] -> Sum4/2
  [dsplay] -> Gain23/1
  Sum1/1 -> [dsplay]  "splay velocity"
  Sum2/1 -> [splay]  "splay angle"
  phi_thigh [rad]/1 -> Sum2/2, [thigh]
  phi_shin [rad]/1 -> Sum2/1, [shin]
  dphi_thigh [rad/s]/1 -> Sum1/2, [dthigh]
  dphi_shin [rad/s]/1 -> Sum1/1, [dshin]
  Mux9/1 -> R PD Torques/4

== system atrias_boom_nmStand_fullCtrl/Control/Behavior Control/Add Limit Avoidance PD Torques/mechanical limit avoidance/PD Joint Limit/R Scale desired torque ==
  note: NOTE: min_splay_angle does not equal delta_phi_min
  phi_thigh [rad] : Inport
  phi_shin [rad] : Inport  Port=2
  Constant : Constant
  Constant1 : Constant  Value=delta_phi_max - delta_phi_max_buffer
  Constant10 : Constant  Value=phi_thigh_max_dropoff
  Constant11 : Constant  Value=phi_shin_min_dropoff
  Constant12 : Constant  Value=phi_shin_max_dropoff
  Constant13 : Constant
  Constant2 : Constant  Value=phi_thigh_max - phi_thigh_max_buffer
  Constant3 : Constant  Value=min_splay_angle+min_splay_buffer
  Constant4 : Constant  Value=phi_thigh_min + phi_thigh_min_buffer
  Constant5 : Constant  Value=phi_shin_max - phi_shin_max_buffer
  Constant6 : Constant  Value=phi_shin_min + phi_shin_min_buffer
  Constant7 : Constant  Value=min_splay_dropoff
  Constant8 : Constant  Value=delta_phi_max_dropoff
  Constant9 : Constant  Value=phi_thigh_min_dropoff
  Divide{,1..5} (6 alike) : Product  Inputs=/*
  Gain : Gain  Gain=-1
  Gain1 : Gain  Gain=-1
  Gain2 : Gain  Gain=-1
  Mux{,1,7..8} (4 alike) : Mux  Inputs=2
  R PD scale : Scope  NumInputPorts=4
      settings: ShowLegends=on  TimeRange=2.5  YMin=-100~-5e+07~-1e+07~-5  YMax=100~1e+07~5e+07~5  SaveName=ScopeData5
  Sum : Sum  Inputs=|+-
  Sum1 : Sum  Inputs=-+|
  Sum2 : Sum  Inputs=+-
  Sum{3..8} (6 alike) : Sum  Inputs=+-|
  [0,1]{,1..5} (6 alike) : Saturate  UpperLimit=1  LowerLimit=0
  max : MinMax  Function=max  Inputs=4
  max2 : MinMax  Function=max  Inputs=4
  scale_back : Outport
  scale_front : Outport  Port=2
  wires:
  phi_shin [rad]/1 -> [shin], Sum2/1
  phi_thigh [rad]/1 -> [thigh], Sum2/2
  Sum2/1 -> [splay]  "splay angle"
  [splay] -> Sum4/2
  Constant3/1 -> Sum4/1
  [splay] -> Sum3/2
  Constant1/1 -> Sum3/1
  [thigh] -> Sum6/2
  Constant4/1 -> Sum6/1
  [thigh] -> Sum5/2
  Constant2/1 -> Sum5/1
  [shin] -> Sum8/2
  Constant6/1 -> Sum8/1
  [shin] -> Sum7/2
  Constant5/1 -> Sum7/1
  [min_thigh_scale] -> Mux/1  "min_thigh_trq"
  [max_thigh_scale] -> Mux/2  "max_thigh_trq"
  Mux/1 -> R PD scale/1
  [min_shin_scale] -> Mux8/1  "min_shin_trq"
  [max_shin_scale] -> Mux8/2  "max_shin_trq"
  Mux8/1 -> R PD scale/2
  Mux7/1 -> R PD scale/3
  [min_splay_scale] -> Mux7/1  "min_splay_trq"
  [max_splay_scale] -> Mux7/2  "max_splay_trq"
  Sum/1 -> Mux1/1, scale_back/1
  Constant/1 -> Sum/1
  max/1 -> Sum/2
  Constant7/1 -> Divide/1
  Sum4/1 -> Divide/2
  Divide/1 -> "[0,1]"/1
  "[0,1]"/1 -> [min_splay_scale]
  Divide1/1 -> "[0,1]1"/1
  "[0,1]1"/1 -> [max_splay_scale]
  Sum3/1 -> Gain/1
  Constant8/1 -> Divide1/1
  Gain/1 -> Divide1/2
  Divide2/1 -> "[0,1]2"/1
  "[0,1]2"/1 -> [min_thigh_scale]
  Sum6/1 -> Divide2/2
  Constant9/1 -> Divide2/1
  Divide3/1 -> "[0,1]3"/1
  "[0,1]3"/1 -> [max_thigh_scale]
  Gain1/1 -> Divide3/2
  Sum5/1 -> Gain1/1
  Constant10/1 -> Divide3/1
  Divide4/1 -> "[0,1]4"/1
  "[0,1]4"/1 -> [min_shin_scale]
  Sum8/1 -> Divide4/2
  Constant11/1 -> Divide4/1
  Divide5/1 -> "[0,1]5"/1
  "[0,1]5"/1 -> [max_shin_scale]
  Sum7/1 -> Gain2/1
  Constant12/1 -> Divide5/1
  Gain2/1 -> Divide5/2
  Constant13/1 -> Sum1/2
  max2/1 -> Sum1/1
  [min_shin_scale] -> max/1
  [max_shin_scale] -> max/2
  [min_splay_scale] -> max2/1, max/3
  [max_splay_scale] -> max2/2, max/4
  [max_thigh_scale] -> max2/4
  [min_thigh_scale] -> max2/3
  Sum1/1 -> Mux1/2, scale_front/1
  Mux1/1 -> R PD scale/4

== system atrias_boom_nmStand_fullCtrl/Control/Behavior Control/Virtual Neuromuscular Control/Muscle Layer/GLU/BE force-length relation ==
  note: Buffer Elasticity BE
  lce [lopt] : Inport
  Constant1 : Constant  Value=1-w
  Math Function : Math  Operator=square  SaturateOnIntegerOverflow=on
  Mux1 : Mux  Inputs=2
  Sum4 : Sum  Inputs=|+-  SaturateOnIntegerOverflow=on  InputSameDT=on  OutDataTypeStr=Inherit: Same as first input
  force above slack length : Fcn  Expr=u(2)*(u(1)<0)
  reference strain [lslack] : Constant  Value=w/2
  relative strain : Product  Inputs=*/
  fbe [Fmax] : Outport
  wires:
  lce [lopt]/1 -> Sum4/1
  Mux1/1 -> force above slack length/1
  force above slack length/1 -> fbe [Fmax]/1
  Math Function/1 -> Mux1/2
  relative strain/1 -> Math Function/1
  reference strain [lslack]/1 -> relative strain/2
  Sum4/1 -> relative strain/1, Mux1/1
  Constant1/1 -> Sum4/2

== system atrias_boom_nmStand_fullCtrl/Control/Behavior Control/Virtual Neuromuscular Control/Muscle Layer/GLU/CE force-length relation ==
  note: CE Force-Length Relationship
  lce [lopt] : Inport
  Abs : Abs
  Constant1 : Constant
  Constant2 : Constant  Value=3
  Gain : Gain  Gain=log(c)
  Math Function : Math  SaturateOnIntegerOverflow=on
  Math Function1 : Math  Operator=pow  SaturateOnIntegerOverflow=on
  Sum4 : Sum  Inputs=|+-  SaturateOnIntegerOverflow=on  InputSameDT=on  OutDataTypeStr=Inherit: Same as first input
  normalized position : Product  Inputs=*/
  relative width : Constant  Value=w
  fce [Fmax] : Outport
  wires:
  lce [lopt]/1 -> Sum4/1
  relative width/1 -> normalized position/2
  Constant1/1 -> Sum4/2
  Sum4/1 -> Abs/1
  Abs/1 -> normalized position/1
  normalized position/1 -> Math Function1/1
  Constant2/1 -> Math Function1/2
  Math Function1/1 -> Gain/1
  Gain/1 -> Math Function/1
  Math Function/1 -> fce [Fmax]/1

== system atrias_boom_nmStand_fullCtrl/Control/Behavior Control/Virtual Neuromuscular Control/Muscle Layer/GLU/CE inverse force-velocity relation ==
  note: CE Inverse Force-Velocity Relationship
  Fv[Fmax] : Inport
  1 : Product  Inputs=/*
  Constant{1,3..4,8} (4 alike) : Constant
  Constant2 : Constant  Value=N
  Constant5 : Constant  Value=N
  Curvature : Gain  Gain=K  SaturateOnIntegerOverflow=on  OutDataTypeStr=Inherit: Same as input  ParamDataTypeStr=Inherit: Same as input
  Curvature1 : Gain  Gain=7.56*K  SaturateOnIntegerOverflow=on  OutDataTypeStr=Inherit: Same as input  ParamDataTypeStr=Inherit: Same as input
  Mux : Mux  Inputs=2
  Mux1 : Mux  Inputs=3
  Mux2 : Mux  Inputs=3
  Slope : Gain  Gain=1e-2  SaturateOnIntegerOverflow=on  OutDataTypeStr=Inherit: Same as input  ParamDataTypeStr=Inherit: Same as input
  Sum1 : Sum  Inputs=|++  SaturateOnIntegerOverflow=on  InputSameDT=on  OutDataTypeStr=Inherit: Same as first input
  Sum2 : Sum  SaturateOnIntegerOverflow=on  InputSameDT=on  OutDataTypeStr=Inherit: Same as first input
  Sum3 : Sum  Inputs=++|  SaturateOnIntegerOverflow=on  InputSameDT=on  OutDataTypeStr=Inherit: Same as first input
  Sum4 : Sum  Inputs=|+-  SaturateOnIntegerOverflow=on  InputSameDT=on  OutDataTypeStr=Inherit: Same as first input
  Sum5 : Sum  Inputs=|-+  SaturateOnIntegerOverflow=on  InputSameDT=on  OutDataTypeStr=Inherit: Same as first input
  Sum6 : Sum  Inputs=-+|  SaturateOnIntegerOverflow=on  InputSameDT=on  OutDataTypeStr=Inherit: Same as first input
  Sum7 : Sum  Inputs=|++  SaturateOnIntegerOverflow=on  InputSameDT=on  OutDataTypeStr=Inherit: Same as first input
  Sum8 : Sum  Inputs=+-|  SaturateOnIntegerOverflow=on  InputSameDT=on  OutDataTypeStr=Inherit: Same as first input
  Sum9 : Sum  SaturateOnIntegerOverflow=on  InputSameDT=on  OutDataTypeStr=Inherit: Same as first input
  concentric branch : Fcn  Expr=u(1) * (u(2)<=1)
  excentric branch : Fcn  Expr=u(2) * (u(1)>1)*(u(1)<=u(3))
  excentric overshoot : Fcn  Expr=u(3) * (u(2)>u(1))
  v_concentric : Product  Inputs=*/
  v_excentric <N : Product  Inputs=*/
  v[vmax] : Outport
  wires:
  Curvature/1 -> Sum3/2
  Constant1/1 -> Sum4/2, Sum3/1
  Sum4/1 -> v_concentric/1
  Sum3/1 -> v_concentric/2
  1/1 -> Sum7/1, Curvature1/1
  Constant4/1 -> Sum7/2, Sum8/1
  Curvature1/1 -> Sum8/2
  Sum8/1 -> v_excentric <N/2
  Sum7/1 -> v_excentric <N/1
  v_concentric/1 -> Mux/1
  Fv[Fmax]/1 -> Sum4/1, Curvature/1, Sum6/2, Mux/2, Mux1/1, Mux2/2
  Sum9/1 -> v[vmax]/1
  Sum2/1 -> Sum9/2
  excentric overshoot/1 -> Sum2/2
  Slope/1 -> Sum1/1
  Constant8/1 -> Sum1/2
  Sum6/1 -> 1/2, Slope/1
  Constant2/1 -> Sum6/1, Sum5/2
  Sum5/1 -> 1/1
  Constant3/1 -> Sum5/1
  Mux/1 -> concentric branch/1
  Mux1/1 -> excentric branch/1
  v_excentric <N/1 -> Mux1/2
  Mux2/1 -> excentric overshoot/1
  concentric branch/1 -> Sum9/1
  excentric branch/1 -> Sum2/1
  Constant5/1 -> Mux1/3, Mux2/1
  Sum1/1 -> Mux2/3

== system atrias_boom_nmStand_fullCtrl/Control/Behavior Control/Virtual Neuromuscular Control/Muscle Layer/GLU/PE force-length relation ==
  note: Parallel Elasticity PE
  lce [lopt] : Inport
  Constant3 : Constant
  Math Function2 : Math  Operator=square  SaturateOnIntegerOverflow=on
  Mux : Mux  Inputs=2
  Sum1 : Sum  Inputs=|+-  SaturateOnIntegerOverflow=on  InputSameDT=on  OutDataTypeStr=Inherit: Same as first input
  force above slack length : Fcn  Expr=u(2) * (u(1)>1)
  reference strain [lopt] : Constant  Value=w
  relative strain : Product  Inputs=*/
  fpe [Fmax] : Outport
  wires:
  Mux/1 -> force above slack length/1
  lce [lopt]/1 -> Mux/1, Sum1/1
  Constant3/1 -> Sum1/2
  Sum1/1 -> relative strain/1
  reference strain [lopt]/1 -> relative strain/2
  relative strain/1 -> Math Function2/1
  Math Function2/1 -> Mux/2
  force above slack length/1 -> fpe [Fmax]/1

== system atrias_boom_nmStand_fullCtrl/Control/Behavior Control/Virtual Neuromuscular Control/Muscle Layer/GLU/SE force-length relation ==
  note: SE Force-Length Relationship
  lse [lslack] : Inport
  Constant1 : Constant
  Math Function : Math  Operator=square  SaturateOnIntegerOverflow=on
  Mux : Mux  Inputs=2
  Sum4 : Sum  Inputs=|+-  SaturateOnIntegerOverflow=on  InputSameDT=on  OutDataTypeStr=Inherit: Same as first input
  force above slack length : Fcn  Expr=u(2)*(u(1)>1)
  reference strain [lslack] : Constant  Value=eref
  relative strain : Product  Inputs=*/
  fse [Fmax] : Outport
  wires:
  Mux/1 -> force above slack length/1
  force above slack length/1 -> fse [Fmax]/1
  Math Function/1 -> Mux/2
  lse [lslack]/1 -> Mux/1, Sum4/1
  relative strain/1 -> Math Function/1
  reference strain [lslack]/1 -> relative strain/2
  Sum4/1 -> relative strain/1
  Constant1/1 -> Sum4/2

== system atrias_boom_nmStand_fullCtrl/Control/Behavior Control/Virtual Neuromuscular Control/Muscle Layer/GLU1/BE force-length relation ==
  note: Buffer Elasticity BE
  lce [lopt] : Inport
  Constant1 : Constant  Value=1-w
  Math Function : Math  Operator=square  SaturateOnIntegerOverflow=on
  Mux1 : Mux  Inputs=2
  Sum4 : Sum  Inputs=|+-  SaturateOnIntegerOverflow=on  InputSameDT=on  OutDataTypeStr=Inherit: Same as first input
  force above slack length : Fcn  Expr=u(2)*(u(1)<0)
  reference strain [lslack] : Constant  Value=w/2
  relative strain : Product  Inputs=*/
  fbe [Fmax] : Outport
  wires:
  lce [lopt]/1 -> Sum4/1
  Mux1/1 -> force above slack length/1
  force above slack length/1 -> fbe [Fmax]/1
  Math Function/1 -> Mux1/2
  relative strain/1 -> Math Function/1
  reference strain [lslack]/1 -> relative strain/2
  Sum4/1 -> relative strain/1, Mux1/1
  Constant1/1 -> Sum4/2

== system atrias_boom_nmStand_fullCtrl/Control/Behavior Control/Virtual Neuromuscular Control/Muscle Layer/GLU1/CE force-length relation ==
  note: CE Force-Length Relationship
  lce [lopt] : Inport
  Abs : Abs
  Constant1 : Constant
  Constant2 : Constant  Value=3
  Gain : Gain  Gain=log(c)
  Math Function : Math  SaturateOnIntegerOverflow=on
  Math Function1 : Math  Operator=pow  SaturateOnIntegerOverflow=on
  Sum4 : Sum  Inputs=|+-  SaturateOnIntegerOverflow=on  InputSameDT=on  OutDataTypeStr=Inherit: Same as first input
  normalized position : Product  Inputs=*/
  relative width : Constant  Value=w
  fce [Fmax] : Outport
  wires:
  lce [lopt]/1 -> Sum4/1
  relative width/1 -> normalized position/2
  Constant1/1 -> Sum4/2
  Sum4/1 -> Abs/1
  Abs/1 -> normalized position/1
  normalized position/1 -> Math Function1/1
  Constant2/1 -> Math Function1/2
  Math Function1/1 -> Gain/1
  Gain/1 -> Math Function/1
  Math Function/1 -> fce [Fmax]/1
